simulink model "Part1sim"  (R2016b)
settings: Solver=VariableStepAuto  StartTime=0.0  StopTime=100.0  RelTol=1e-3
settings Model: Creator=Alex  LastModifiedBy=Alex

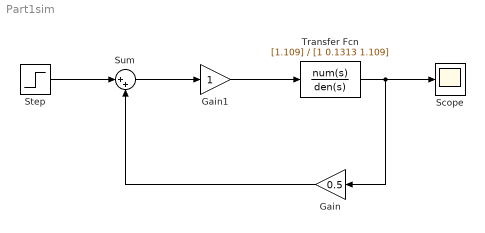
== system Part1sim ==
  Gain : Gain  Gain=0.5
  Gain1 : Gain
  Scope : Scope
  Step : Step  SampleTime=0
  Sum : Sum  Inputs=|++
  Transfer Fcn : TransferFcn  Numerator=[1.109]  Denominator=[1 0.1313 1.109]
  wires:
  Step/1 -> Sum/1
  Gain/1 -> Sum/2
  Transfer Fcn/1 -> Gain/1, Scope/1
  Gain1/1 -> Transfer Fcn/1
  Sum/1 -> Gain1/1
